simulink model "DP_controller"  (R2019a)
settings: Solver=VariableStepAuto  StartTime=0.0  StopTime=10.0  RelTol=1e-3
undefined symbols (not defined in the file or in its folder): Kd1, Kd2, Kd3, Ki1, Ki2, Ki3, Kp1, Kp2, Kp3
settings Model: Creator=den  LastModifiedBy=den

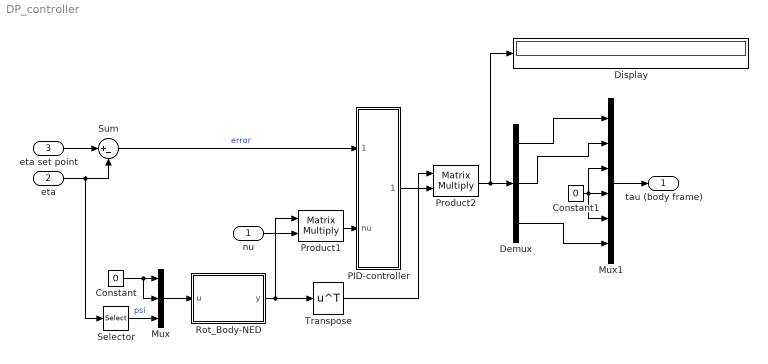
== system DP_controller ==
  nu : Inport
  eta : Inport  Port=2
  eta set point : Inport  Port=3
  Constant : Constant  Value=0
  Constant1 : Constant  Value=0
  Demux : Demux  Outputs=3
  Display : Display
  Mux : Mux  Inputs=3
  Mux1 : Mux  Inputs=6
  PID-controller : Subsystem  mask{Kp=[Kp1 Kp2 Kp3], Ki=[Ki1 Ki2 Ki3], Kd=[Kd1 Kd2 Kd3]}
  Product1 : Product  Multiplication=Matrix(*)
  Product2 : Product  Multiplication=Matrix(*)
  Rot_Body-NED : MATLAB Function  TreatAsAtomicUnit=on
  Selector : Selector  InputPortWidth=3  IndexOptions=Index vector (dialog)  Indices=[3]  OutputSizes=1
  Sum : Sum  Inputs=|+-
  Transpose : Math  Operator=transpose  SaturateOnIntegerOverflow=on
  tau (body frame) : Outport
  wires:
  Constant1/1 -> Mux1/3, Mux1/5, Mux1/4
  Mux1/1 -> tau (body frame)/1
  Product1/1 -> PID-controller/2(nu)
  Sum/1 -> PID-controller/1(error)  "error"
  Constant/1 -> Mux/2, Mux/1
  eta/1 -> Selector/1, Sum/2
  Product2/1 -> Display/1, Demux/1
  Mux/1 -> Rot_Body-NED/1(u)
  nu/1 -> Product1/2
  PID-controller/1(tau) -> Product2/2
  eta set point/1 -> Sum/1
  Demux/3 -> Mux1/6
  Rot_Body-NED/1(y) -> Transpose/1, Product1/1
  Selector/1 -> Mux/3  "psi"
  Transpose/1 -> Product2/1
  Demux/1 -> Mux1/1
  Demux/2 -> Mux1/2

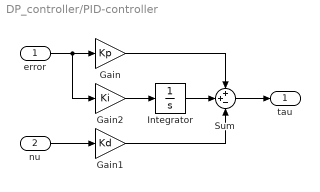
== system DP_controller/PID-controller ==
  error : Inport
  nu : Inport  Port=2
  Gain : Gain  Gain=Kp
  Gain1 : Gain  Gain=Kd
  Gain2 : Gain  Gain=Ki
  Integrator : Integrator  LimitOutput=on  UpperSaturationLimit=[8e5 8e5 2e6]  LowerSaturationLimit=-[8e5 8e5 2e6]
  Sum : Sum  Inputs=++-
  tau : Outport
  wires:
  Gain1/1 -> Sum/3
  Gain/1 -> Sum/1
  nu/1 -> Gain1/1
  error/1 -> Gain2/1, Gain/1
  Integrator/1 -> Sum/2
  Sum/1 -> tau/1
  Gain2/1 -> Integrator/1

== matlab function DP_controller/Rot_Body-NED ==
  data: u input; y output
function y = rot_zyx(u)
% Rzyx: Available in the MSS-toolbox
y = Rzyx(u(1), u(2), u(3));
